simulink model "TurtleBotFeedbackLinearizationSimulation"  (R2022b)
settings: Solver=VariableStepAuto  StartTime=0.0  StopTime=45  RelTol=1e-8  AbsTol=1e-8
settings Model: Creator=gianm  LastModifiedBy=aless

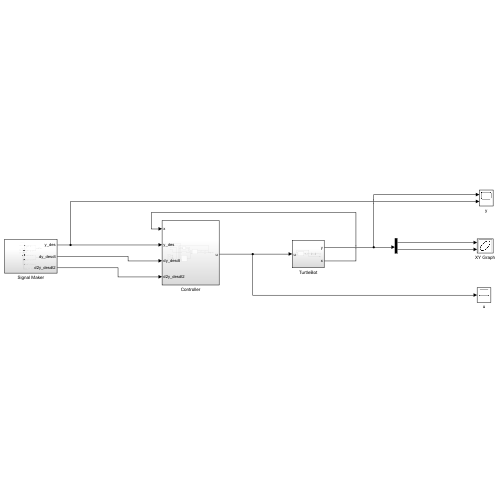
[thumbnail: Simulink's stored preview of the top-level diagram]
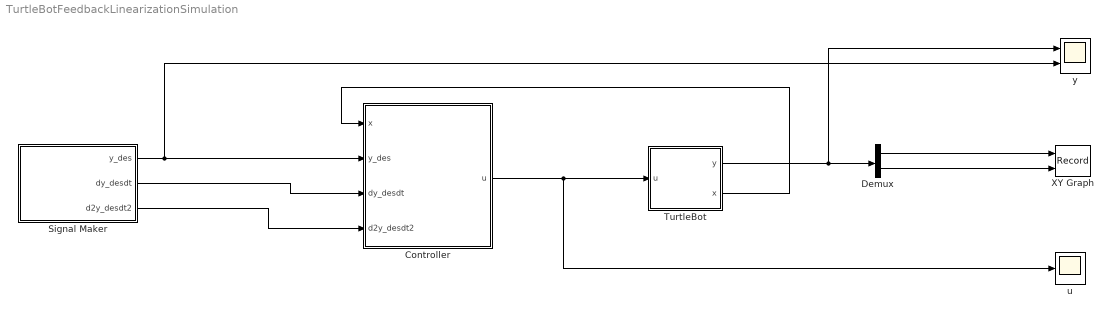
== system TurtleBotFeedbackLinearizationSimulation ==
  Controller : Subsystem
  Demux : Demux  Outputs=2
  Signal Maker : Subsystem
  TurtleBot : Subsystem
  XY Graph : Record  FileSettingsInternal="{\"entries\":[{\"content\":{\"excelSettings\":{\"content\":{},\"type\":\"Streamout.ExcelSettings\"}},\"type\":\"Streamout.FileSettingStorage\",\"uuid\":\"\"}],\"packageUris\":[\"http:\\/\\/schema.mathworks.com\\/mf0\\/streamout_blocks\\/R2020a\"],\"version\":\"1.0\"}"  Layout=[1 1]  SignalsInternal="{\"entries\":[{\"content\":{\"signals\":[{\"content\":{\"blockPath\":[],\"channel\":[],\"dimensions\":[1],\"domain\":\"\",\"lineColor\":\"#edb120\",\"plots\":[1],\"port\":1,\"sid\":[\"\"],\"signalID\":395,\"signalName\":\"Demux:1\"},\"type\":\"RecordBlkView.Signal\",\"uuid\":\"\"},{\"content\":{\"blockPath\":[],\"channel\":[],\"dimensions\":[1],\"domain\":\"\",\"lineColor\":\"#7e2f8e\",\"plots\":[1],\"port\":2,\"sid\":[\"\"],\"signalID\":399,\"signalName\":\"Demux:2\"},\"type\":\"RecordBlkView.Signal\",\"uuid\":\"\"}]},\"type\":\"RecordBlkView.InputSignals\",\"uuid\":\"\"}],\"packageUris\":[\"http:\\/\\/schema.mathworks.com\\/mf0\\/streamout_blocks\\/R2020a\"],\"version\":\"1.0\"}"  VisualizationBindings="{\"xyplotplugin\":{\"info\":[{\"series\":[{\"bindingParametersList\":[{\"parameter\":\"X-Axis\",\"signalID\":395,\"signalName\":\"Demux:1\"},{\"parameter\":\"Y-Axis\",\"signalID\":399,\"signalName\":\"Demux:2\"}],\"seriesID\":65267}],\"subplotID\":1}]}}"  CompatibilityTag=XY
  u : Scope
  y : Scope  NumInputPorts=2
  wires:
  TurtleBot/1(y) -> y/1, Demux/1
  Demux/1 -> XY Graph/1
  Demux/2 -> XY Graph/2
  Signal Maker/1(y_des) -> y/2, Controller/2(y_des)
  TurtleBot/2(x) -> Controller/1(x)
  Signal Maker/2(dy_desdt) -> Controller/3(dy_desdt)
  Controller/1(u) -> u/1, TurtleBot/1(u)
  Signal Maker/3(d2y_desdt2) -> Controller/4(d2y_desdt2)

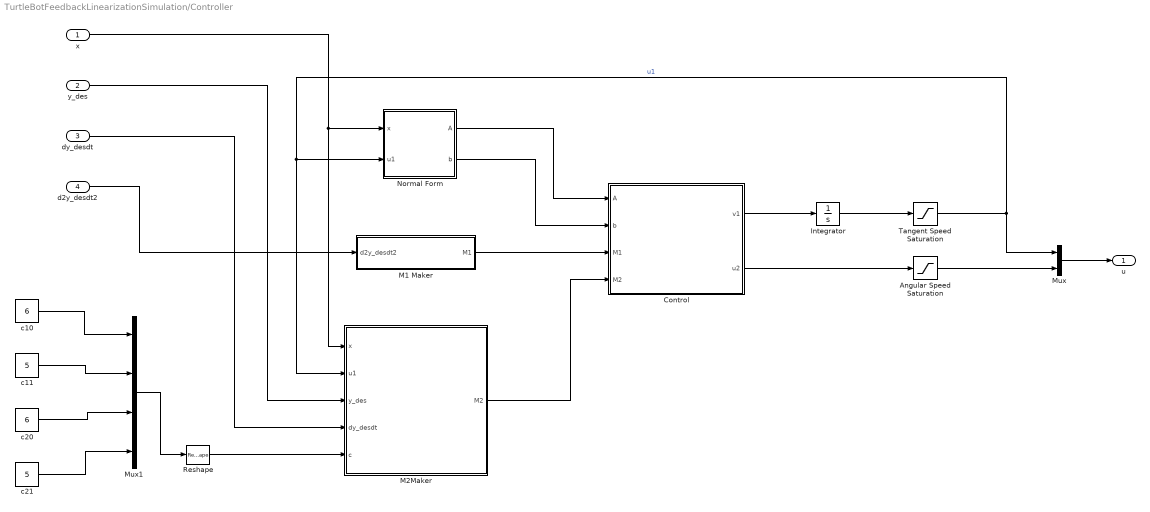
== system TurtleBotFeedbackLinearizationSimulation/Controller ==
  x : Inport
  y_des : Inport  Port=2
  dy_desdt : Inport  Port=3
  d2y_desdt2 : Inport  Port=4
  Angular Speed Saturation : Saturate  UpperLimit=0.8  LowerLimit=-0.8
  Control : MATLAB Function  TreatAsAtomicUnit=on
  Integrator : Integrator  InitialCondition=0.01
  M1 Maker : Subsystem
  M2Maker : MATLAB Function  TreatAsAtomicUnit=on
  Mux : Mux  Inputs=2
  Mux1 : Mux
  Normal Form : MATLAB Function  TreatAsAtomicUnit=on
  Reshape : Reshape  OutputDimensionality=Column vector (2-D)
  Tangent Speed Saturation : Saturate  UpperLimit=0.1  LowerLimit=-0.1
  c10 : Constant  Value=6
  c11 : Constant  Value=5
  c20 : Constant  Value=6
  c21 : Constant  Value=5
  u : Outport
  wires:
  y_des/1 -> M2Maker/3(y_des)
  Normal Form/1(A) -> Control/1(A)
  M1 Maker/1(M1) -> Control/3(M1)
  Control/1(v1) -> Integrator/1
  x/1 -> Normal Form/1(x), M2Maker/1(x)
  Control/2(u2) -> Angular Speed Saturation/1
  Integrator/1 -> Tangent Speed Saturation/1
  Mux/1 -> u/1
  dy_desdt/1 -> M2Maker/4(dy_desdt)
  d2y_desdt2/1 -> M1 Maker/1(d2y_desdt2)
  Normal Form/2(b) -> Control/2(b)
  M2Maker/1(M2) -> Control/4(M2)
  Mux1/1 -> Reshape/1
  c21/1 -> Mux1/4
  c20/1 -> Mux1/3
  c10/1 -> Mux1/1
  c11/1 -> Mux1/2
  Reshape/1 -> M2Maker/5(c)
  Tangent Speed Saturation/1 -> Normal Form/2(u1), M2Maker/2(u1), Mux/1  "u1"
  Angular Speed Saturation/1 -> Mux/2

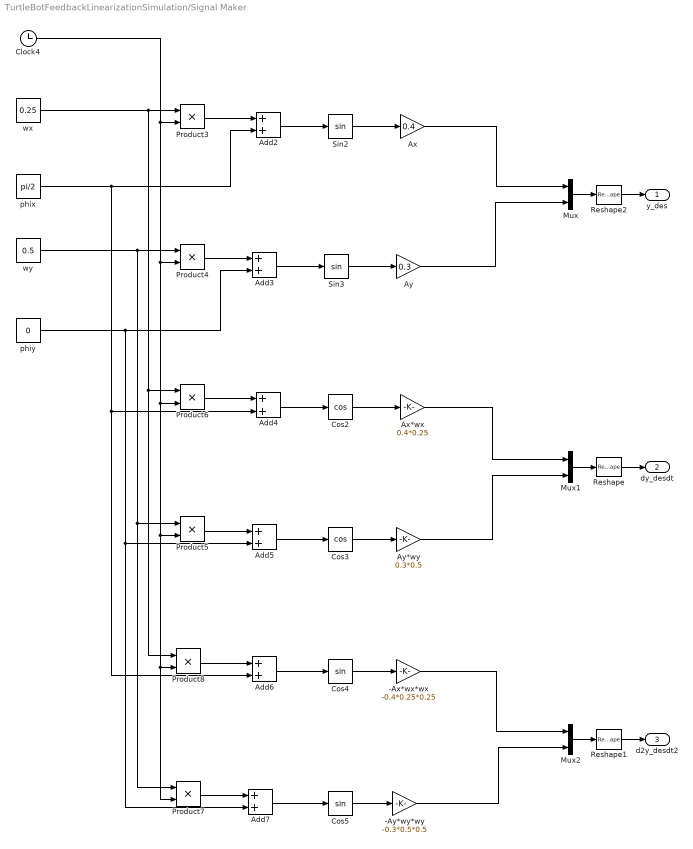
== system TurtleBotFeedbackLinearizationSimulation/Signal Maker ==
  -Ax*wx*wx : Gain  Gain=-0.4*0.25*0.25
  -Ay*wy*wy : Gain  Gain=-0.3*0.5*0.5
  Add{2..7} (6 alike) : Sum
  Ax : Gain  Gain=0.4
  Ax*wx : Gain  Gain=0.4*0.25
  Ay : Gain  Gain=0.3
  Ay*wy : Gain  Gain=0.3*0.5
  Clock4 : Clock
  Cos2 : Trigonometry  Operator=cos
  Cos3 : Trigonometry  Operator=cos
  Cos4 : Trigonometry
  Cos5 : Trigonometry
  Mux : Mux  Inputs=2
  Mux1 : Mux  Inputs=2
  Mux2 : Mux  Inputs=2
  Product{3..8} (6 alike) : Product
  Reshape : Reshape  OutputDimensionality=Column vector (2-D)
  Reshape1 : Reshape  OutputDimensionality=Column vector (2-D)
  Reshape2 : Reshape  OutputDimensionality=Column vector (2-D)
  Sin2 : Trigonometry
  Sin3 : Trigonometry
  phix : Constant  Value=pi/2
  phiy : Constant  Value=0
  wx : Constant  Value=0.25
  wy : Constant  Value=0.5
  y_des : Outport
  dy_desdt : Outport  Port=2
  d2y_desdt2 : Outport  Port=3
  wires:
  Ax/1 -> Mux/1
  Reshape2/1 -> y_des/1
  Ay*wy/1 -> Mux1/2
  Reshape1/1 -> d2y_desdt2/1
  Product7/1 -> Add7/1
  Cos4/1 -> -Ax*wx*wx/1
  Add6/1 -> Cos4/1
  -Ay*wy*wy/1 -> Mux2/2
  Product6/1 -> Add4/1
  Add4/1 -> Cos2/1
  Mux1/1 -> Reshape/1
  Add5/1 -> Cos3/1
  Product4/1 -> Add3/1
  wy/1 -> Product7/1, Product5/1, Product4/1
  phix/1 -> Add6/2, Add4/2, Add2/2
  -Ax*wx*wx/1 -> Mux2/1
  Clock4/1 -> Product7/2, Product8/2, Product5/2, Product6/2, Product4/2, Product3/2
  Add2/1 -> Sin2/1
  Mux2/1 -> Reshape1/1
  Ax*wx/1 -> Mux1/1
  Sin2/1 -> Ax/1
  Ay/1 -> Mux/2
  Product3/1 -> Add2/1
  Cos2/1 -> Ax*wx/1
  wx/1 -> Product8/1, Product6/1, Product3/1
  Add3/1 -> Sin3/1
  phiy/1 -> Add7/2, Add5/2, Add3/2
  Product8/1 -> Add6/1
  Add7/1 -> Cos5/1
  Cos5/1 -> -Ay*wy*wy/1
  Sin3/1 -> Ay/1
  Reshape/1 -> dy_desdt/1
  Product5/1 -> Add5/1
  Cos3/1 -> Ay*wy/1
  Mux/1 -> Reshape2/1

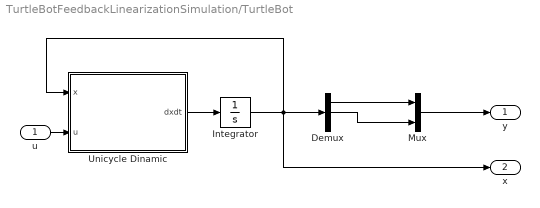
== system TurtleBotFeedbackLinearizationSimulation/TurtleBot ==
  u : Inport
  Demux : Demux  Outputs=3
  Integrator : Integrator  InitialCondition=[0;0;0]
  Mux : Mux  Inputs=2
  Unicycle Dinamic : MATLAB Function  TreatAsAtomicUnit=on
  y : Outport
  x : Outport  Port=2
  wires:
  Unicycle Dinamic/1(dxdt) -> Integrator/1
  Integrator/1 -> x/1, Demux/1, Unicycle Dinamic/1(x)
  u/1 -> Unicycle Dinamic/2(u)
  Demux/1 -> Mux/1
  Demux/2 -> Mux/2
  Mux/1 -> y/1

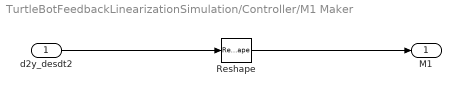
== system TurtleBotFeedbackLinearizationSimulation/Controller/M1 Maker ==
  d2y_desdt2 : Inport
  Reshape : Reshape  OutputDimensionality=Column vector (2-D)
  M1 : Outport
  wires:
  d2y_desdt2/1 -> Reshape/1
  Reshape/1 -> M1/1

== matlab function TurtleBotFeedbackLinearizationSimulation/Controller/Control ==
  data: A input; b input; M1 input; v1 output; M2 input; u2 output
function [v1, u2] = control(A, b, M1, M2)

    u = inv(A)*(-b + M1 + M2);

    v1 = u(1);
    u2 = u(2);
    
end

== matlab function TurtleBotFeedbackLinearizationSimulation/TurtleBot/Unicycle Dinamic ==
  data: x input; dxdt output; u input
function dxdt = P(x, u)

    dxdt = [cos(x(3))*u(1);
            sin(x(3))*u(1);
            u(2)];
    
end

== matlab function TurtleBotFeedbackLinearizationSimulation/Controller/Normal Form ==
  data: x input; A output; u1 input; b output
function [A, b] = normalForm(x, u1)
    
    A = [cos(x(3)), -u1*sin(x(3));
        sin(x(3)),  u1*cos(x(3))];
    
    b = [0;
         0];
    
end

== matlab function TurtleBotFeedbackLinearizationSimulation/Controller/M2Maker ==
  data: x input; u1 input; y_des input; dy_desdt input; c input; M2 output
function M2 = M2Maker(x, u1, y_des, dy_desdt, c)

    M2 = [-c(1)*(x(1) - y_des(1)) - c(2)*(u1*cos(x(3)) - dy_desdt(1));
          -c(3)*(x(2) - y_des(2)) - c(4)*(u1*sin(x(3)) - dy_desdt(2))];

end
